simulink model "kalman_filter"  (Simulink 7.7)
settings: Solver=ode45  StartTime=0.0  StopTime=10.0  RelTol=1e-3
libraries: UAVdesign_net x1
settings Model: Creator=Emanuel  LastModifiedBy=Emanuel
settings DebuggingCC: StrictBusMsg=Warning
settings SFSimCC: SimParseCustomCode=off

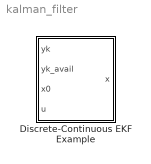
== system kalman_filter ==
  Discrete-Continuous EKF Example : Subsystem

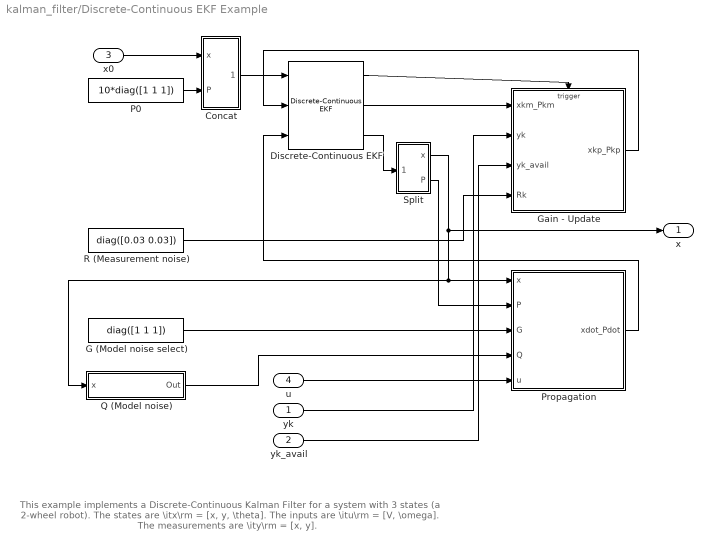
== system kalman_filter/Discrete-Continuous EKF Example ==
  note: This example implements a Discrete-Continuous Kalman Filter
      | for a system with 3 states (a 2-wheel robot).
      | The states are \itx\rm = [x, y, \theta].
      | The inputs are \itu\rm = [V, \omega].
      | The measurements are \ity\rm = [x, y].
  yk : Inport
  yk_avail : Inport  Port=2
  x0 : Inport  Port=3
  u : Inport  Port=4
  Concat : Subsystem
  Discrete-Continuous EKF : UAVdesign_net/Utilities/Kalman Filter/Discrete-Continuous EKF  sample_time=1
  G (Model noise select) : Constant  Value=diag([1 1 1])
  Gain - Update : Subsystem  TreatAsAtomicUnit=on
  P0 : Constant  Value=10*diag([1 1 1])
  Propagation : Subsystem
  Q (Model noise) : Subsystem
  R (Measurement noise) : Constant  Value=diag([0.03 0.03])
  Split : Subsystem
  x : Outport
  wires:
  Discrete-Continuous EKF/2 -> Gain - Update/1(xkm_Pkm)
  Discrete-Continuous EKF/3 -> Split/1(x_P)
  Propagation/1(xdot_Pdot) -> Discrete-Continuous EKF/3
  Concat/1(x_P) -> Discrete-Continuous EKF/1
  P0/1 -> Concat/2(P)
  x0/1 -> Concat/1(x)
  Gain - Update/1(xkp_Pkp) -> Discrete-Continuous EKF/2
  Split/2(P) -> Propagation/2(P)
  G (Model noise select)/1 -> Propagation/3(G)
  Q (Model noise)/1(Out) -> Propagation/4(Q)
  R (Measurement noise)/1 -> Gain - Update/4(Rk)
  Discrete-Continuous EKF/1 -> Gain - Update/Trigger
  yk/1 -> Gain - Update/2(yk)
  yk_avail/1 -> Gain - Update/3(yk_avail)
  Split/1(x) -> x/1, Propagation/1(x), Q (Model noise)/1(x)
  u/1 -> Propagation/5(u)

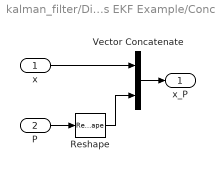
== system kalman_filter/Discrete-Continuous EKF Example/Concat ==
  x : Inport
  P : Inport  Port=2
  Reshape : Reshape
  Vector Concatenate : Concatenate  Mode=Vector
  x_P : Outport
  wires:
  P/1 -> Reshape/1
  Vector Concatenate/1 -> x_P/1
  x/1 -> Vector Concatenate/1
  Reshape/1 -> Vector Concatenate/2

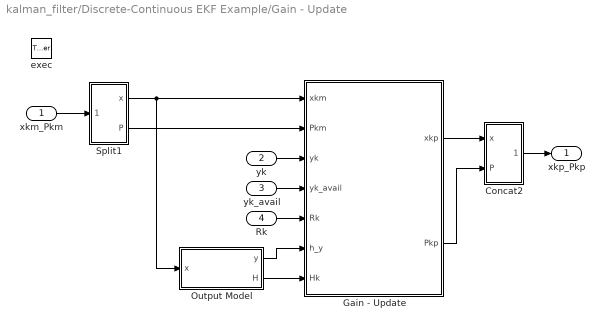
== system kalman_filter/Discrete-Continuous EKF Example/Gain - Update ==
  xkm_Pkm : Inport
  yk : Inport  Port=2
  yk_avail : Inport  Port=3
  Rk : Inport  Port=4
  exec : TriggerPort  TriggerType=function-call
  Concat2 : Subsystem
  Gain - Update : Stateflow chart  TreatAsAtomicUnit=on
  Output Model : Subsystem
  Split1 : Subsystem
  xkp_Pkp : Outport
  wires:
  Output Model/1(y) -> Gain - Update/6(h_y)
  Output Model/2(H) -> Gain - Update/7(Hk)
  Rk/1 -> Gain - Update/5(Rk)
  yk_avail/1 -> Gain - Update/4(yk_avail)
  Split1/2(P) -> Gain - Update/2(Pkm)
  yk/1 -> Gain - Update/3(yk)
  Split1/1(x) -> Gain - Update/1(xkm), Output Model/1(x)
  xkm_Pkm/1 -> Split1/1(x_P)
  Gain - Update/1(xkp) -> Concat2/1(x)
  Gain - Update/2(Pkp) -> Concat2/2(P)
  Concat2/1(x_P) -> xkp_Pkp/1

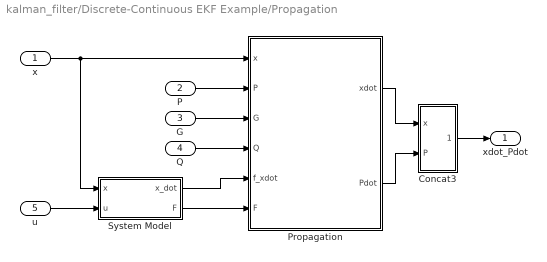
== system kalman_filter/Discrete-Continuous EKF Example/Propagation ==
  x : Inport
  P : Inport  Port=2
  G : Inport  Port=3
  Q : Inport  Port=4
  u : Inport  Port=5
  Concat3 : Subsystem
  Propagation : Stateflow chart  TreatAsAtomicUnit=on
  System Model : Subsystem
  xdot_Pdot : Outport
  wires:
  u/1 -> System Model/2(u)
  System Model/1(x_dot) -> Propagation/5(f_xdot)
  Q/1 -> Propagation/4(Q)
  x/1 -> System Model/1(x), Propagation/1(x)
  P/1 -> Propagation/2(P)
  G/1 -> Propagation/3(G)
  System Model/2(F) -> Propagation/6(F)
  Concat3/1(x_P) -> xdot_Pdot/1
  Propagation/1(xdot) -> Concat3/1(x)
  Propagation/2(Pdot) -> Concat3/2(P)

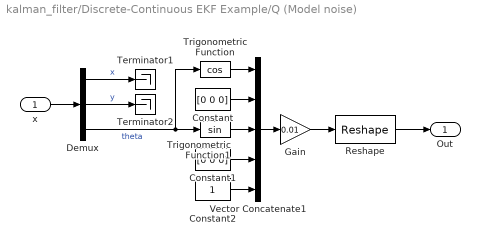
== system kalman_filter/Discrete-Continuous EKF Example/Q (Model noise) ==
  x : Inport
  Constant : Constant  Value=[0 0 0]
  Constant1 : Constant  Value=[0 0 0]
  Constant2 : Constant
  Demux : Demux  Outputs=3
  Gain : Gain  Gain=0.01
  Reshape : Reshape  OutputDimensionality=Customize  OutputDimensions=[3,3]
  Terminator1 : Terminator
  Terminator2 : Terminator
  Trigonometric Function : Trigonometry  Operator=cos
  Trigonometric Function1 : Trigonometry
  Vector Concatenate1 : Concatenate  NumInputs=5  Mode=Vector
  Out : Outport
  wires:
  Reshape/1 -> Out/1
  Vector Concatenate1/1 -> Gain/1
  Constant/1 -> Vector Concatenate1/2
  Constant1/1 -> Vector Concatenate1/4
  Gain/1 -> Reshape/1
  Constant2/1 -> Vector Concatenate1/5
  Trigonometric Function1/1 -> Vector Concatenate1/3
  Trigonometric Function/1 -> Vector Concatenate1/1
  x/1 -> Demux/1
  Demux/1 -> Terminator1/1  "x"
  Demux/2 -> Terminator2/1  "y"
  Demux/3 -> Trigonometric Function1/1, Trigonometric Function/1  "theta"

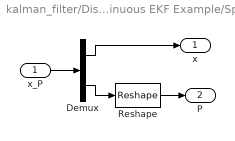
== system kalman_filter/Discrete-Continuous EKF Example/Split ==
  x_P : Inport
  Demux : Demux  Outputs=[3 9]
  Reshape : Reshape  OutputDimensionality=Customize  OutputDimensions=[3,3]
  x : Outport
  P : Outport  Port=2
  wires:
  Reshape/1 -> P/1
  x_P/1 -> Demux/1
  Demux/1 -> x/1
  Demux/2 -> Reshape/1

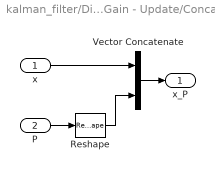
== system kalman_filter/Discrete-Continuous EKF Example/Gain - Update/Concat2 ==
  x : Inport
  P : Inport  Port=2
  Reshape : Reshape
  Vector Concatenate : Concatenate  Mode=Vector
  x_P : Outport
  wires:
  P/1 -> Reshape/1
  Vector Concatenate/1 -> x_P/1
  x/1 -> Vector Concatenate/1
  Reshape/1 -> Vector Concatenate/2

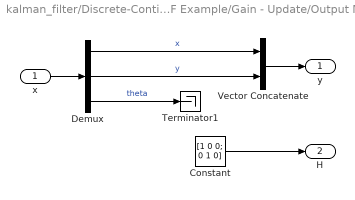
== system kalman_filter/Discrete-Continuous EKF Example/Gain - Update/Output Model ==
  x : Inport
  Constant : Constant  Value=[1 0 0; 0 1 0]
  Demux : Demux  Outputs=3
  Terminator1 : Terminator
  Vector Concatenate : Concatenate  Mode=Vector
  y : Outport
  H : Outport  Port=2
  wires:
  Demux/1 -> Vector Concatenate/1  "x"
  Demux/2 -> Vector Concatenate/2  "y"
  Demux/3 -> Terminator1/1  "theta"
  x/1 -> Demux/1
  Vector Concatenate/1 -> y/1
  Constant/1 -> H/1

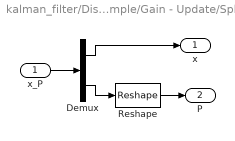
== system kalman_filter/Discrete-Continuous EKF Example/Gain - Update/Split1 ==
  x_P : Inport
  Demux : Demux  Outputs=[3 9]
  Reshape : Reshape  OutputDimensionality=Customize  OutputDimensions=[3,3]
  x : Outport
  P : Outport  Port=2
  wires:
  Reshape/1 -> P/1
  x_P/1 -> Demux/1
  Demux/1 -> x/1
  Demux/2 -> Reshape/1

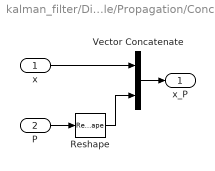
== system kalman_filter/Discrete-Continuous EKF Example/Propagation/Concat3 ==
  x : Inport
  P : Inport  Port=2
  Reshape : Reshape
  Vector Concatenate : Concatenate  Mode=Vector
  x_P : Outport
  wires:
  Reshape/1 -> Vector Concatenate/2
  x/1 -> Vector Concatenate/1
  Vector Concatenate/1 -> x_P/1
  P/1 -> Reshape/1

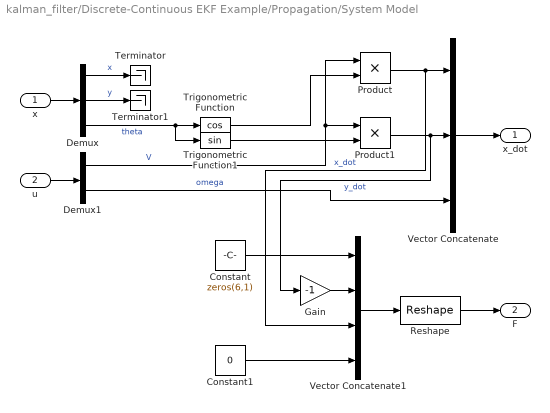
== system kalman_filter/Discrete-Continuous EKF Example/Propagation/System Model ==
  x : Inport
  u : Inport  Port=2
  Constant : Constant  Value=zeros(6,1)
  Constant1 : Constant  Value=0
  Demux : Demux  Outputs=3
  Demux1 : Demux  Outputs=2
  Gain : Gain  Gain=-1
  Product : Product  RndMeth=Zero
  Product1 : Product  RndMeth=Zero
  Reshape : Reshape  OutputDimensionality=Customize  OutputDimensions=[3,3]
  Terminator : Terminator
  Terminator1 : Terminator
  Trigonometric Function : Trigonometry  Operator=cos
  Trigonometric Function1 : Trigonometry
  Vector Concatenate : Concatenate  NumInputs=3  Mode=Vector
  Vector Concatenate1 : Concatenate  NumInputs=4  Mode=Vector
  x_dot : Outport
  F : Outport  Port=2
  wires:
  Vector Concatenate/1 -> x_dot/1
  x/1 -> Demux/1
  Demux/1 -> Terminator/1  "x"
  Demux/2 -> Terminator1/1  "y"
  Demux/3 -> Trigonometric Function/1, Trigonometric Function1/1  "theta"
  u/1 -> Demux1/1
  Demux1/1 -> Product/1, Product1/1  "V"
  Demux1/2 -> Vector Concatenate/3  "omega"
  Trigonometric Function/1 -> Product/2
  Product/1 -> Vector Concatenate/1, Vector Concatenate1/3  "x_dot"
  Trigonometric Function1/1 -> Product1/2
  Product1/1 -> Vector Concatenate/2, Gain/1  "y_dot"
  Reshape/1 -> F/1
  Vector Concatenate1/1 -> Reshape/1
  Constant/1 -> Vector Concatenate1/1
  Gain/1 -> Vector Concatenate1/2
  Constant1/1 -> Vector Concatenate1/4

== matlab function Discrete-Continuous EKF Example/Gain - Update/Gain - Update ==
  data: xkm input double; Pkm input double; yk input double; yk_avail input double; Rk input double; h_y input double; Hk input double; xkp output double; Pkp output double
function [xkp, Pkp] = EKF_d(xkm, Pkm, yk, yk_avail, Rk, h_y, Hk)

Nx = length(xkm);
Ny = length(yk);
    
% Make sure P is symmetric and well-behaved
Pkm = (Pkm + Pkm') / 2;
for i=1:Nx
    if Pkm(i,i) <= 0
        Pkm(i,i) = 1e-10;
    end
end

if sum(yk_avail) > 0
    % Measurements are available. Construct the h matrix.
    y_small = zeros(Ny,1);
    h_small = zeros(Ny,1);
    H_small = zeros(Ny, Nx);
    R_small = eye(Ny, Ny);
    
    index = 0;
    for i=1:Ny
        if yk_avail(i)
            index = index+1;
            y_small(index) = yk(i);
            h_small(index) = h_y(i);
            H_small(index, :) = Hk(i, :);
            index2 = 0;
            for j=1:Ny
                if yk_avail(j)
                    index2 = index2+1;
                    R_small(index, index2) = Rk(i, j);
                end
            end
        end
    end
    
%    index = Ny;
%    y_small = yk;
%    h_small = h_y;
%    H_small = Hk;
%    R_small = Rk;
    
    % Gain
    inv_temp = inv(H_small * Pkm * H_small' + R_small);
    if index < Ny
        for i=(index+1):Ny
            inv_temp(i,:) = zeros(1, Ny);
            inv_temp(:,i) = zeros(Ny, 1);
        end
    end
    Kk = Pkm * H_small' * inv_temp;

    % Update
    xkp = xkm + Kk * (y_small - h_small);
    Pkp = (eye(Nx, Nx) - Kk * H_small) * Pkm;
else
    % No measurements available
    xkp = xkm;
    Pkp = Pkm;
end

% Make sure P is symmetric and well-behaved
Pkp = (Pkp + Pkp') / 2;
for i=1:Nx
    if Pkp(i,i) <= 0
        Pkp(i,i) = 1e-10;
    end
end

== matlab function Discrete-Continuous EKF Example/Propagation/Propagation ==
  data: x input double; P input double; G input double; Q input double; f_xdot input double; F input double; xdot output double; Pdot output double
function [xdot, Pdot] = EKF_c(x, P, G, Q, f_xdot, F)

Nx = length(x);

xdot = f_xdot;
Pdot = F * P + P * F' + G * Q * G';
